simulink model "engine_model_test_221218"  (R2018b)
settings: Solver=ode14x  StartTime=0.0  StopTime=10.0  FixedStep=0.005  RelTol=1e-3
values from neighbouring files (symbols this model uses):
  F = 5e-5    (= 5e-05)    [BLDC_simulator.m]    (also in engine_parameters.m; engine_parameters_20191210.m = 1)
  J = 7.22e-6    (= 7.22e-06)    [BLDC_simulator.m]    (also in IMU.m = [cos(theta_2)*cos(theta_3) sin(theta_3) 0; engine_parameters.m; engine_parameters_20191210.m = 0.001)
  Kt = 8.44e-3    (= 0.00844)    [BLDC_simulator.m]    (also in engine_parameters.m)
  Kv = 8.44e-3    (= 0.00844)    [BLDC_simulator.m]    (also in engine_parameters.m)
  L = 0.42e-3    (= 0.00042)    [BLDC_simulator.m]    (also in engine_parameters.m; engine_parameters_20191210.m = 0.0005)
  R = 7.9    [BLDC_simulator.m]    (also in engine_parameters.m; engine_parameters_20191210.m = 0.5; inversekinematics.m = Rg*Rd*Rm)
undefined symbols (not defined in the file or in its folder): sigbuilder_block
libraries: simulink x5, simulink_extras x3
settings Model: Creator=Paweł Tymiński  LastModifiedBy=Paweł Tymiński

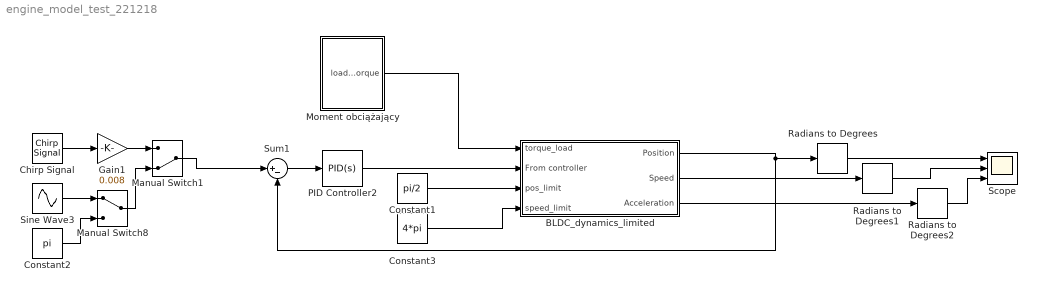
== system engine_model_test_221218 ==
  BLDC_dynamics_limited : Subsystem
  Chirp Signal : simulink/Sources/Chirp Signal  f1=1  T=20  f2=10
  Constant1 : Constant  Value=pi/2
  Constant2 : Constant  Value=pi
  Constant3 : Constant  Value=4*pi
  Gain1 : Gain  Gain=0.008
  Manual Switch1 : ManualSwitch  CurrentSetting=0
  Manual Switch8 : ManualSwitch
  Moment obciążający : Subsystem
  PID Controller2 : simulink/Continuous/PID Controller  Controller=PID  Form=Ideal  TimeDomain=Continuous-time  SampleTime=-1  IntegratorMethod=Forward Euler  FilterMethod=Forward Euler  ControllerParametersSource=internal  P=5.17125627242477  I=0.879628779481434  D=0.157743378330372  UseFilter=on  N=13783.089028979  TunerSelectOption=Transfer Function Based (PID Tuner App)  InitialConditionSource=internal  InitialConditionForIntegrator=0  InitialConditionForFilter=0  DifferentiatorICPrevScaledInput=0  ExternalReset=none  TrackingMode=off  Kt=1  LimitOutput=off  UpperSaturationLimit=inf  LowerSaturationLimit=-inf  LinearizeAsGain=on  AntiWindupMode=none  Kb=1  POutMin=[]  POutMax=[]  IOutMin=[]  IOutMax=[]  DOutMin=[]  DOutMax=[]  NOutMin=[]  NOutMax=[]  SumOutMin=[]  SumOutMax=[]  SaturationOutMin=[]  SaturationOutMax=[]  PParamMin=[]  PParamMax=[]  IParamMin=[]  IParamMax=[]  DParamMin=[]  DParamMax=[]  NParamMin=[]  NParamMax=[]  KbParamMin=[]  KbParamMax=[]  KtParamMin=[]  KtParamMax=[]  KbOutMin=[]  KbOutMax=[]  KtOutMin=[]  KtOutMax=[]  IntegratorOutMin=[]  IntegratorOutMax=[]  FilterOutMin=[]  FilterOutMax=[]  SumI1OutMin=[]  SumI1OutMax=[]  SumI2OutMin=[]  SumI2OutMax=[]  SumI3OutMin=[]  SumI3OutMax=[]  SumI4OutMin=[]  SumI4OutMax=[]  SumDOutMin=[]  SumDOutMax=[]  DifferentiatorOutMin=[]  DifferentiatorOutMax=[]  FilterDiffOutCoefMin=[]  FilterDiffOutCoefMax=[]  ReciprocalOutMin=[]  ReciprocalOutMax=[]  SumDenOutMin=[]  SumDenOutMax=[]  SumNumOutMin=[]  SumNumOutMax=[]  DivideOutMin=[]  DivideOutMax=[]  IntegratorContinuousStateAttributes=''  IntegratorStateMustResolveToSignalObject=off  IntegratorRTWStateStorageClass=Auto  FilterContinuousStateAttributes=''  FilterStateMustResolveToSignalObject=off  FilterRTWStateStorageClass=Auto  ParallelPVariant=Passthrough  IdealPVariant=InternalParameters  IVariant=InternalParameters  DVariant=InternalParameters  IntegratorVariant=Continuous  SatVariant=Disabled  AWVariant=Passthrough  PCopyVariant=Disabled  TRVariant=Disabled  FdbkBlocksVariant=Forward  IdealPFdbkVariant=Disabled  SatFdbkVariant=Disabled  DerivativeFilterVariant=ContFilter  NVariant=InternalParameters  NCopyVariant=Disabled  FilterICVariant=InternalICsFilter  IntegratorICVariant=InternalICs  ExternalResetVariant=Disabled  TRSumVariant=Passthrough  SumFdbkVariant=Disabled  SumVariant=Sum_PID
  Radians to Degrees : simulink_extras/Transformations/Radians to Degrees
  Radians to Degrees1 : simulink_extras/Transformations/Radians to Degrees
  Radians to Degrees2 : simulink_extras/Transformations/Radians to Degrees
  Scope : Scope  NumInputPorts=3
  Sine Wave3 : Sin  Amplitude=pi  Frequency=2*pi  SampleTime=0
  Sum1 : Sum  Inputs=|+-
  wires:
  Manual Switch8/1 -> Manual Switch1/2
  Sum1/1 -> PID Controller2/1
  BLDC_dynamics_limited/1(Position) -> Radians to Degrees/1, Sum1/2
  Moment obciążający/1(load_torque) -> BLDC_dynamics_limited/1(torque_load)
  Constant2/1 -> Manual Switch8/2
  PID Controller2/1 -> BLDC_dynamics_limited/2(From controller)
  Constant3/1 -> BLDC_dynamics_limited/4(speed_limit)
  Constant1/1 -> BLDC_dynamics_limited/3(pos_limit)
  Sine Wave3/1 -> Manual Switch8/1
  Gain1/1 -> Manual Switch1/1
  Chirp Signal/1 -> Gain1/1
  Manual Switch1/1 -> Sum1/1
  BLDC_dynamics_limited/2(Speed) -> Radians to Degrees1/1
  BLDC_dynamics_limited/3(Acceleration) -> Radians to Degrees2/1
  Radians to Degrees/1 -> Scope/1
  Radians to Degrees2/1 -> Scope/3
  Radians to Degrees1/1 -> Scope/2

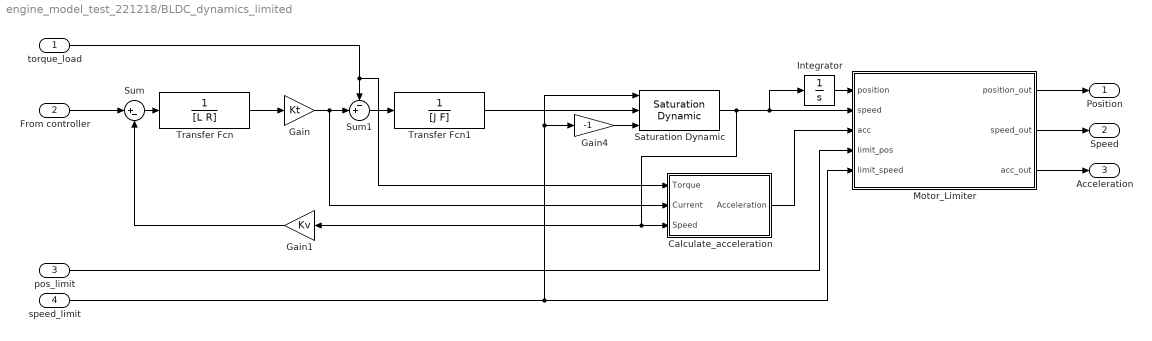
== system engine_model_test_221218/BLDC_dynamics_limited ==
  torque_load : Inport
  From controller : Inport  Port=2
  pos_limit : Inport  Port=3
  speed_limit : Inport  Port=4
  Calculate_acceleration : Subsystem
  Gain : Gain  Gain=Kt
  Gain1 : Gain  Gain=Kv
  Gain4 : Gain  Gain=-1
  Integrator : Integrator
  Motor_Limiter : MATLAB Function  TreatAsAtomicUnit=on
  Saturation Dynamic : simulink/Discontinuities/Saturation Dynamic  OutMin=[]  OutMax=[]  OutDataTypeStr=Inherit: Same as second input  OutDataType=fixdt(1, 16)  OutScaling=2^-10  DoSatur=off
  Sum : Sum  Inputs=|+-
  Sum1 : Sum  Inputs=-+|
  Transfer Fcn : TransferFcn  Denominator=[L R]
  Transfer Fcn1 : TransferFcn  Denominator=[J F]
  Position : Outport
  Speed : Outport  Port=2
  Acceleration : Outport  Port=3
  wires:
  Gain/1 -> Calculate_acceleration/2(Current), Sum1/2
  Transfer Fcn/1 -> Gain/1
  Sum/1 -> Transfer Fcn/1
  From controller/1 -> Sum/1
  torque_load/1 -> Calculate_acceleration/1(Torque), Sum1/1
  Gain1/1 -> Sum/2
  Sum1/1 -> Transfer Fcn1/1
  Transfer Fcn1/1 -> Saturation Dynamic/2
  Saturation Dynamic/1 -> Calculate_acceleration/3(Speed), Gain1/1, Motor_Limiter/2(speed), Integrator/1
  Gain4/1 -> Saturation Dynamic/3
  Motor_Limiter/1(position_out) -> Position/1
  Motor_Limiter/2(speed_out) -> Speed/1
  Motor_Limiter/3(acc_out) -> Acceleration/1
  Calculate_acceleration/1(Acceleration) -> Motor_Limiter/3(acc)
  Integrator/1 -> Motor_Limiter/1(position)
  speed_limit/1 -> Motor_Limiter/5(limit_speed), Saturation Dynamic/1, Gain4/1
  pos_limit/1 -> Motor_Limiter/4(limit_pos)

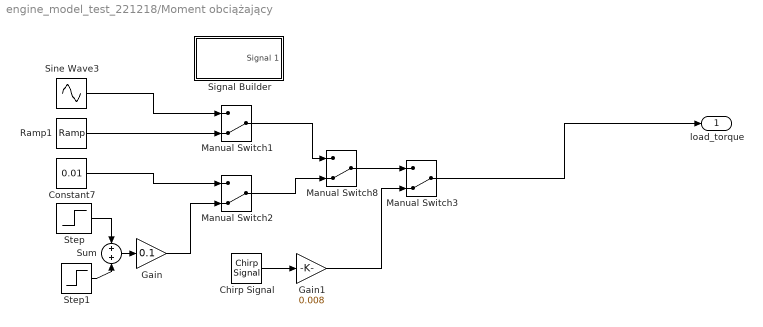
== system engine_model_test_221218/Moment obciążający ==
  Chirp Signal : simulink/Sources/Chirp Signal  f1=1  T=20  f2=10
  Constant7 : Constant  Value=0.01
  Gain : Gain  Gain=0.1
  Gain1 : Gain  Gain=0.008
  Manual Switch{1..3,8} (4 alike) : ManualSwitch  CurrentSetting=0
  Ramp1 : simulink/Sources/Ramp  slope=pi/16  start=0  InitialOutput=0
  Signal Builder : Subsystem  Tag=STV Subsys  LoadFcn=sigbuilder_block('load');  StartFcn=sigbuilder_block('start');  StopFcn=sigbuilder_block('stop');  ClipboardFcn=sigbuilder_block('clipboard');  mask(Sigbuilder block){tuvar=[0:10]}
      mask help: Simulink:masks:SigbuilderBlock_MD
      mask init:
      | if ~strcmp(get_param(bdroot(gcbh),'SimulationStatus'),'stopped') tuvar = sigbuilder_block('maskInit'); end
      settings: CopyFcn=sigbuilder_block('copy');  DeleteFcn=sigbuilder_block('delete');  ModelCloseFcn=sigbuilder_block('modelClose');  PreSaveFcn=sigbuilder_block('preSave');  PauseFcn=sigbuilder_block('pause');  ContinueFcn=sigbuilder_block('continue');  NameChangeFcn=sigbuilder_block('namechange');  OpenFcn=sigbuilder_block('open',[437.6 199.2 550.4 400 ]);  CloseFcn=sigbuilder_block('close');
      mask Display: plot(0, 0, 100, 100,[2, 2, 32, 32, 2], [68, 8, 8, 68, 68],[32, 2], [38, 38], [32, 19, 2],[53, 60, 44], [32, 17, 17, 2],[16, 16, 31, 31]);txt = getActiveGroup(gcbh);text(2, 100, txt,'verticalAlignment', 'top');
  Sine Wave3 : Sin  Amplitude=pi/18  SampleTime=0
  Step : Step  SampleTime=0
  Step1 : Step  Time=2  After=-1  SampleTime=0
  Sum : Sum
  load_torque : Outport
  wires:
  Step/1 -> Sum/1
  Constant7/1 -> Manual Switch2/1
  Gain/1 -> Manual Switch2/2
  Step1/1 -> Sum/2
  Sine Wave3/1 -> Manual Switch1/1
  Manual Switch1/1 -> Manual Switch8/1
  Manual Switch2/1 -> Manual Switch8/2
  Sum/1 -> Gain/1
  Ramp1/1 -> Manual Switch1/2
  Chirp Signal/1 -> Gain1/1
  Manual Switch3/1 -> load_torque/1
  Manual Switch8/1 -> Manual Switch3/1
  Gain1/1 -> Manual Switch3/2

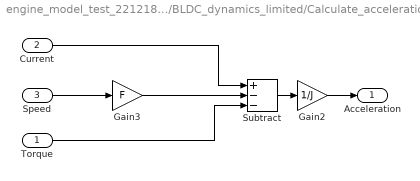
== system engine_model_test_221218/BLDC_dynamics_limited/Calculate_acceleration ==
  Torque : Inport
  Current : Inport  Port=2
  Speed : Inport  Port=3
  Gain2 : Gain  Gain=1/J
  Gain3 : Gain  Gain=F
  Subtract : Sum  Inputs=+--
  Acceleration : Outport
  wires:
  Gain3/1 -> Subtract/2
  Subtract/1 -> Gain2/1
  Gain2/1 -> Acceleration/1
  Current/1 -> Subtract/1
  Speed/1 -> Gain3/1
  Torque/1 -> Subtract/3

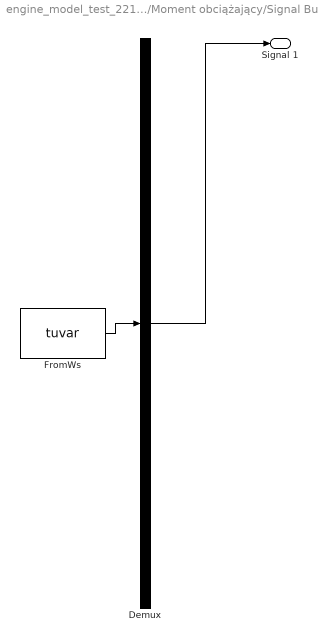
== system engine_model_test_221218/Moment obciążający/Signal Builder ==
  Demux : Demux  Tag=STV Demux  Outputs=1
  FromWs : FromWorkspace  Tag=STV FromWs  VariableName=tuvar  SampleTime=0
      SigBuilderData=|
      | common.afterFinalStr = 'Extrapolate'
      | common.sampleTime = 0
      | dataSet.timeRange = [0 10]
      | dataSet.name = 'Group 1'
      | sbobj.Groups.Name = 'Group 1'
      | sbobj.Groups.Signals.Name = 'Signal 1'
      | sbobj.Groups.Signals.XData = [0 4 4 6 6 10]
      | sbobj.Groups.Signals.YData = [-0.015 0.125 0.575 0.895 0.04 0]
  Signal 1 : Outport  Tag=STV Outport
  wires:
  Demux/1 -> Signal 1/1
  FromWs/1 -> Demux/1

== matlab function engine_model_test_221218/BLDC_dynamics_limited/Motor_Limiter ==
  data: position input; position_out output; speed input; speed_out output; acc input; limit_pos input; limit_speed input; acc_out output
function [position_out,speed_out,acc_out] = fcn(position, speed,  acc, limit_pos, limit_speed)
if abs(position)>=limit_pos  & abs(speed) >= limit_speed
	position_out=sign(position)*limit_pos;
	speed_out=0;
	acc_out=0;
elseif abs(position)>=limit_pos  & abs(speed) <= limit_speed
	position_out=sign(position)*limit_pos;
	speed_out=0;
	acc_out=0;	
elseif	abs(position)<=limit_pos  & abs(speed) >= limit_speed
	position_out=position;
	speed_out=sign(speed)*limit_speed;
	acc_out=0;	
else 	
    position_out=position;
    speed_out=speed;
    acc_out=acc;
end
